simulink model "Fig36"  (Simulink 8.4)
settings: Solver=ode3  StartTime=0.0  StopTime=5.24288  FixedStep=2e-6  RelTol=1e-5
libraries: commchan3 x1, commrandsrc2 x1
settings Model: Creator=Dennis Silage  LastModifiedBy=Silage
settings OptimizationCC: InitFltsAndDblsToZero=on
settings DebuggingCC: SolverPrmCheckMsg=none

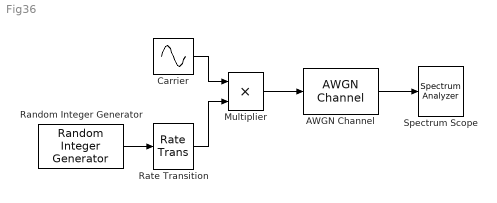
== system Fig36 ==
  AWGN Channel : commchan3/AWGN Channel  InputProcessing=Inherited (this choice will be removed - see release notes)  seed=randseed  noiseMode=Variance from mask  EbNodB=80  EsNodB=10  SNRdB=10  bitsPerSym=1  Ps=25  Tsym=1e-3  variance=0
  Carrier : Sin  Amplitude=5  Frequency=40000*pi  SampleTime=2e-6
  "Multiplier " : Product  RndMeth=Zero
  Random Integer Generator : commrandsrc2/Random Integer Generator  mul=2  seed=randseed  Ts=1e-3  frameBased=off  sampPerFrame=50  orient=on  outDataType=double
  Rate Transition : RateTransition  OutPortSampleTime=2e-6
  Spectrum Scope : SpectrumAnalyzer
  wires:
  Random Integer Generator/1 -> Rate Transition/1
  "Multiplier "/1 -> AWGN Channel/1
  Rate Transition/1 -> "Multiplier "/2
  Carrier/1 -> "Multiplier "/1
  AWGN Channel/1 -> Spectrum Scope/1
